simulink model "bitToInteger"  (R2020b)
settings: Solver=VariableStepAuto  StartTime=0.0  StopTime=10.0  RelTol=1e-3
libraries: commutil2 x1
settings Model: Creator=yinti  LastModifiedBy=yinti

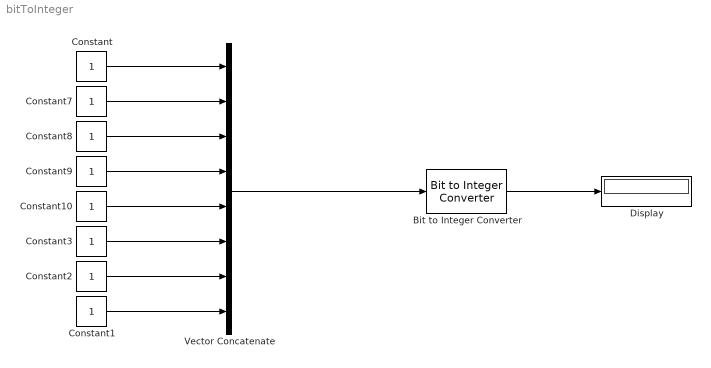
== system bitToInteger ==
  Bit to Integer Converter : commutil2/Bit to Integer Converter  nbits=8  bitOrder=LSB first  signedOutputValues=Unsigned  outDtype=Inherit via internal rule  outDtypeSigned=Inherit via internal rule
  Constant{,1..3,7..10} (8 alike) : Constant
  Display : Display
  Vector Concatenate : Concatenate  NumInputs=8
  wires:
  Vector Concatenate/1 -> Bit to Integer Converter/1
  Bit to Integer Converter/1 -> Display/1
  Constant/1 -> Vector Concatenate/1
  Constant1/1 -> Vector Concatenate/8
  Constant2/1 -> Vector Concatenate/7
  Constant3/1 -> Vector Concatenate/6
  Constant7/1 -> Vector Concatenate/2
  Constant8/1 -> Vector Concatenate/3
  Constant9/1 -> Vector Concatenate/4
  Constant10/1 -> Vector Concatenate/5
